simulink model "P702_NI_SoftECU"  (R2019a)
settings: Solver=ode1  StartTime=0.0  StopTime=Inf  FixedStep=0.001  RelTol=1e-3  EnableMultiTasking=on
PreLoadFcn:
  | run '.\VeriStand_BlockSet\NIVeriStandAddPaths.m'
undefined symbols (not defined in the file or in its folder): magnitude
libraries: simulink x83, simulink_extras x1
(part 69 of 76)

== system P702_NI_SoftECU/Output/Subsystem2/To_NI_HIL/Soft_SCCM/Steering_Data ==
  AccButtnGapDecPress : Constant  Value=0
  AccButtnGapIncPress : Constant  Value=0
  AhbStat_B_Dsply : Constant  Value=0
  AslButtnOnOffCnclPress : Constant  Value=0
  AslButtnOnOffPress : Constant  Value=0
  CcAslButtnCnclPress : Constant  Value=0
  CcAslButtnCnclResPress : Constant  Value=0
  CcAslButtnOnPress : Constant  Value=0
  CcAslButtnResDecPress : Constant  Value=0
  CcAslButtnResIncPress : Constant  Value=0
  CcAslButtnSetDecPress : Constant  Value=0
  CcAslButtnSetIncPress : Constant  Value=0
  CcAslButtnSetPress : Constant  Value=0
  CcAsllButtnResPress : Constant  Value=0
  CcButtnOffPress : Constant  Value=0
  CcButtnOnOffCnclPress : Constant  Value=0
  CcButtnOnOffPress : Constant  Value=0
  CcButtnOnPress : Constant  Value=0
  HeadLghtHiCtrl_D_RqAhb : Constant  Value=0
  HeadLghtHiOn_B_StatAhb : Constant  Value=0
  bus_creator : BusCreator  Inputs=20
  out_port : Outport
  wires:
  bus_creator/1 -> out_port/1  "Subsystem2"
  AhbStat_B_Dsply/1 -> bus_creator/1  "AhbStat_B_Dsply"
  HeadLghtHiCtrl_D_RqAhb/1 -> bus_creator/2  "HeadLghtHiCtrl_D_RqAhb"
  HeadLghtHiOn_B_StatAhb/1 -> bus_creator/3  "HeadLghtHiOn_B_StatAhb"
  CcButtnOnPress/1 -> bus_creator/4  "CcButtnOnPress"
  CcButtnOffPress/1 -> bus_creator/5  "CcButtnOffPress"
  CcAslButtnCnclPress/1 -> bus_creator/6  "CcAslButtnCnclPress"
  CcAsllButtnResPress/1 -> bus_creator/7  "CcAsllButtnResPress"
  CcAslButtnResIncPress/1 -> bus_creator/8  "CcAslButtnResIncPress"
  CcAslButtnSetIncPress/1 -> bus_creator/9  "CcAslButtnSetIncPress"
  CcAslButtnSetDecPress/1 -> bus_creator/10  "CcAslButtnSetDecPress"
  CcAslButtnSetPress/1 -> bus_creator/11  "CcAslButtnSetPress"
  AccButtnGapIncPress/1 -> bus_creator/12  "AccButtnGapIncPress"
  AccButtnGapDecPress/1 -> bus_creator/13  "AccButtnGapDecPress"
  AslButtnOnOffPress/1 -> bus_creator/14  "AslButtnOnOffPress"
  AslButtnOnOffCnclPress/1 -> bus_creator/15  "AslButtnOnOffCnclPress"
  CcButtnOnOffPress/1 -> bus_creator/16  "CcButtnOnOffPress"
  CcButtnOnOffCnclPress/1 -> bus_creator/17  "CcButtnOnOffCnclPress"
  CcAslButtnResDecPress/1 -> bus_creator/18  "CcAslButtnResDecPress"
  CcAslButtnOnPress/1 -> bus_creator/19  "CcAslButtnOnPress"
  CcAslButtnCnclResPress/1 -> bus_creator/20  "CcAslButtnCnclResPress"

== system P702_NI_SoftECU/Output/Subsystem2/To_NI_HIL/Soft_SCCM/Steering_Wheel_Data2 ==
  SteWhlSwtchBack_B_Stat : Constant  Value=0
  SteWhlSwtchDown_B_Stat : Constant  Value=0
  SteWhlSwtchLeft_B_Stat : Constant  Value=0
  SteWhlSwtchMenu_B_Stat : Constant  Value=0
  SteWhlSwtchOk_B_Stat : Constant  Value=0
  SteWhlSwtchRght_B_Stat : Constant  Value=0
  SteWhlSwtchUp_B_Stat : Constant  Value=0
  bus_creator : BusCreator  Inputs=7
  out_port : Outport
  wires:
  bus_creator/1 -> out_port/1  "Subsystem2"
  SteWhlSwtchOk_B_Stat/1 -> bus_creator/1  "SteWhlSwtchOk_B_Stat"
  SteWhlSwtchUp_B_Stat/1 -> bus_creator/2  "SteWhlSwtchUp_B_Stat"
  SteWhlSwtchDown_B_Stat/1 -> bus_creator/3  "SteWhlSwtchDown_B_Stat"
  SteWhlSwtchLeft_B_Stat/1 -> bus_creator/4  "SteWhlSwtchLeft_B_Stat"
  SteWhlSwtchRght_B_Stat/1 -> bus_creator/5  "SteWhlSwtchRght_B_Stat"
  SteWhlSwtchMenu_B_Stat/1 -> bus_creator/6  "SteWhlSwtchMenu_B_Stat"
  SteWhlSwtchBack_B_Stat/1 -> bus_creator/7  "SteWhlSwtchBack_B_Stat"

== system P702_NI_SoftECU/Output/Subsystem2/To_NI_HIL/Soft_TCM/TransGearData ==
  GearLvrPos_D_Actl : Constant  Value=0
  bus_creator : BusCreator  Inputs=1
  out_port : Outport
  wires:
  bus_creator/1 -> out_port/1  "Subsystem2"
  GearLvrPos_D_Actl/1 -> bus_creator/1  "GearLvrPos_D_Actl"

== system P702_NI_SoftECU/SoftECU/ABS/Logic/Wheel Direction/If Action Subsystem1 ==
  In1 : Inport
  Action Port : ActionPort  ActionPortLabel=if { }
  Out1 : Outport
  wires:
  In1/1 -> Out1/1

== system P702_NI_SoftECU/SoftECU/ABS/Logic/Wheel Direction/If Action Subsystem2 ==
  In1 : Inport
  Action Port : ActionPort  ActionPortLabel=elseif { }
  Out1 : Outport
  wires:
  In1/1 -> Out1/1

== system P702_NI_SoftECU/SoftECU/ABS/Logic/Wheel Direction/If Action Subsystem3 ==
  In1 : Inport
  Action Port : ActionPort  ActionPortLabel=elseif { }
  Out1 : Outport
  wires:
  In1/1 -> Out1/1

== system P702_NI_SoftECU/SoftECU/ABS/Logic/Wheel Direction/If Action Subsystem4 ==
  In1 : Inport
  Action Port : ActionPort  ActionPortLabel=if { }
  Out1 : Outport
  wires:
  In1/1 -> Out1/1

== system P702_NI_SoftECU/SoftECU/ABS/Logic/Wheel Direction/If Action Subsystem5 ==
  In1 : Inport
  Action Port : ActionPort  ActionPortLabel=elseif { }
  Out1 : Outport
  wires:
  In1/1 -> Out1/1

== system P702_NI_SoftECU/SoftECU/ABS/Logic/Wheel Direction/If Action Subsystem6 ==
  In1 : Inport
  Action Port : ActionPort  ActionPortLabel=elseif { }
  Out1 : Outport
  wires:
  In1/1 -> Out1/1

== system P702_NI_SoftECU/SoftECU/BCM/Logic/IgnitionState/If Action Subsystem1 ==
  In1 : Inport
  Action Port : ActionPort  ActionPortLabel=if { }
  Out1 : Outport
  wires:
  In1/1 -> Out1/1

== system P702_NI_SoftECU/SoftECU/BCM/Logic/IgnitionState/If Action Subsystem2 ==
  In1 : Inport
  Action Port : ActionPort  ActionPortLabel=elseif { }
  Out1 : Outport
  wires:
  In1/1 -> Out1/1

== system P702_NI_SoftECU/SoftECU/BCM/Logic/IgnitionState/If Action Subsystem3 ==
  In1 : Inport
  Action Port : ActionPort  ActionPortLabel=elseif { }
  Out1 : Outport
  wires:
  In1/1 -> Out1/1

== system P702_NI_SoftECU/SoftECU/BCM/Logic/IgnitionState/If Action Subsystem4 ==
  In1 : Inport
  Action Port : ActionPort  ActionPortLabel=elseif { }
  Out1 : Outport
  wires:
  In1/1 -> Out1/1

== system P702_NI_SoftECU/SoftECU/BCM/Logic/IgnitionState/If Action Subsystem5 ==
  In1 : Inport
  Action Port : ActionPort  ActionPortLabel=else { }
  Out1 : Outport
  wires:
  In1/1 -> Out1/1

== system P702_NI_SoftECU/SoftECU/BCM/Logic/OdometerValues/If Action Subsystem1 ==
  In1 : Inport
  Action Port : ActionPort  ActionPortLabel=if { }
  Out1 : Outport
  wires:
  In1/1 -> Out1/1

== system P702_NI_SoftECU/SoftECU/BCM/Logic/OdometerValues/If Action Subsystem4 ==
  In1 : Inport
  Action Port : ActionPort  ActionPortLabel=else { }
  Out1 : Outport
  wires:
  In1/1 -> Out1/1

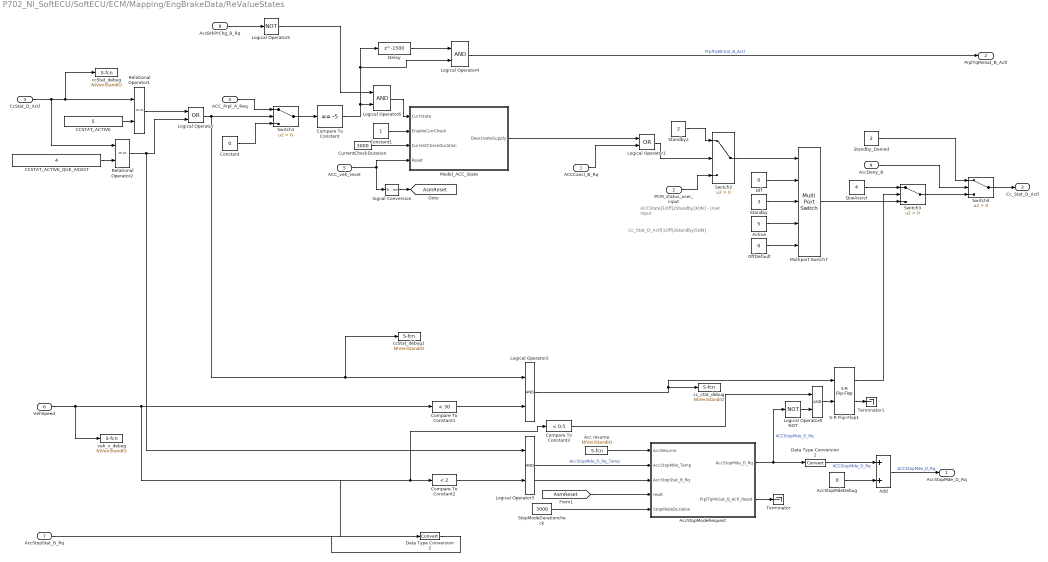
== system P702_NI_SoftECU/SoftECU/ECM/Mapping/EngBrakeData/ReValueStates ==
  note: ACCState[1Off|2Standby|3ON] -
      | User Input
  note: Cc_Stat_D_Actl[1Off|3Standby|5ON]
  ACCCancl_B_Rq : Inport
  PCM_status_user_input : Inport  Port=2
  CcStat_D_Actl : Inport  Port=3
  ACC_Prpl_A_Req : Inport  Port=4
  ACC_veh_reset : Inport  Port=5
  VehSpeed : Inport  Port=6
  AccStopStat_B_Rq : Inport  Port=7
  AccBrkPrChg_B_Rq : Inport  Port=8
  AccDeny_B : Inport  Port=9  OutDataTypeStr=boolean
  Acc resume : S-Function  Priority=1  FunctionName=NIVeriStandIO  Parameters=width dtype portnum stime stype btype  SFunctionDeploymentMode=off  EnableBusSupport=off  mask(NI VeriStand Inport){portnum=1, width=-1, stime=-1, dtype=auto, stype=auto, btype=1}
      mask prompts: portnum "Port number:"; width "Port dimensions (-1 for dynamically sized):"; stime "Sample time (-1 for inherited):"; dtype "Data type:"; stype "Signal type:"; btype "Block type:"
      mask help: Use this inport on any level of nested subsystems to allow NI VeriStand software to map signals to it.
      mask init:
      | NIVeriStandIO_init;
      settings: CopyFcn=NIVeriStand_MDL_functions('', 'IO_copy');  DeleteFcn=NIVeriStand_MDL_functions('', 'IO_delete');  MoveFcn=set_param(gcb, 'Mask', 'on');
      mask Callback portnum: NIVeriStand_MDL_functions('', 'IO_setportnum');
      mask TypeOptions dtype: auto | double | single | int8 | uint8 | int16 | uint16 | int32 | uint32 | boolean
      mask Callback dtype: NIVeriStand_MDL_functions('', 'IO_booleansignal');
      mask TypeOptions stype: auto | real | complex
      mask Display:
      | patch([-x x], [-y y], [.90980 .81960 .32156]);
      | plot([xrad -x x xrad], [yrad -y y yrad]);
      | fprintf('NI In%d', portnum);
  AccStopMdeDebug : Constant  Value=0
  AccStopModeRequest : Stateflow chart  TreatAsAtomicUnit=on
  Active : Constant  Value=5
  Add : Sum  OutDataTypeStr=double
  CCSTAT_ACTIVE : Constant  Description=_V1P2R1PX.CMM.000_81_  Value=5
  CCSTAT_ACTIVE_QUE_ASSIST : Constant  Description=_V1P2R1PX.CMM.000_82_  Value=4
  Compare To Constant : simulink/Logic and Bit Operations/Compare To Constant  relop===  const=-5  OutDataTypeStr=boolean
  Compare To Constant1 : simulink/Logic and Bit Operations/Compare To Constant  relop=<  const=30  OutDataTypeStr=boolean
  Compare To Constant2 : simulink/Logic and Bit Operations/Compare To Constant  relop=<  const=2  OutDataTypeStr=boolean
  Compare To Constant3 : simulink/Logic and Bit Operations/Compare To Constant  relop=<  const=0.5  OutDataTypeStr=boolean
  Constant : Constant  Value=0
  Constant1 : Constant
  CurrentCheckDuration : Constant  Value=3000  OutDataTypeStr=double
  Data Type Conversion1 : DataTypeConversion
  Data Type Conversion2 : DataTypeConversion
  Delay : Delay  DelayLength=1500
  Logical Operator : Logic  Description=_V1P2R1PX.CMM.000_84_  Operator=OR  AllPortsSameDT=off  OutDataTypeStr=boolean
  Logical Operator1 : Logic  Operator=OR  AllPortsSameDT=off  OutDataTypeStr=boolean
  Logical Operator2 : Logic  IconShape=distinctive  AllPortsSameDT=off  OutDataTypeStr=boolean
  Logical Operator3 : Logic  IconShape=distinctive  AllPortsSameDT=off  OutDataTypeStr=boolean
  Logical Operator4 : Logic  AllPortsSameDT=off  OutDataTypeStr=boolean
  Logical Operator5 : Logic  Operator=NOT  AllPortsSameDT=off  OutDataTypeStr=boolean
  Logical Operator6 : Logic  AllPortsSameDT=off  OutDataTypeStr=boolean
  Logical Operator8 : Logic  IconShape=distinctive  AllPortsSameDT=off  OutDataTypeStr=boolean
  Model_ACC_State : Stateflow chart  TreatAsAtomicUnit=on
  Multiport Switch7 : MultiPortSwitch  DataPortForDefault=Additional data port  SaturateOnIntegerOverflow=on
  NOT : Logic  Operator=NOT  IconShape=distinctive  AllPortsSameDT=off  OutDataTypeStr=boolean
  Off : Constant  Value=0
  OffDefault : Constant  Value=0
  QueAssist : Constant  Value=4
  Relational Operator1 : RelationalOperator  Description=_V1P2R1PX.CMM.000_85_  Operator===  OutDataTypeStr=boolean  RndMeth=Nearest
  Relational Operator2 : RelationalOperator  Description=_V1P2R1PX.CMM.000_86_  Operator===  OutDataTypeStr=boolean  RndMeth=Nearest
  S-R Flip-Flop1 : simulink_extras/Flip Flops/S-R Flip-Flop  initial_condition=0
  Signal Conversion : SignalConversion  OverrideOpt=off
  Standby : Constant  Value=3
  Standby2 : Constant  Value=2
  "Standby_Denied " : Constant  Value=2
  StopModeDurationcheck : Constant  Value=3000  OutDataTypeStr=uint16
  Switch{1..4} (4 alike) : Switch  Criteria=u2 > Threshold
  Terminator : Terminator
  Terminator1 : Terminator
  ccStat_debug : S-Function  Priority=3  FunctionName=NIVeriStandIO  Parameters=width dtype portnum stime stype btype  SFunctionDeploymentMode=off  EnableBusSupport=off  mask(NI VeriStand Outport){portnum=3, width=-1, stime=-1, dtype=auto, stype=auto, btype=0}
      mask prompts: portnum "Port number:"; width "Port dimensions (-1 for dynamically sized):"; stime "Sample time (-1 for inherited):"; dtype "Data type:"; stype "Signal type:"; btype "Block type:"
      mask help: Use this outport on any level of nested subsystems to allow NI VeriStand software to map signals to it.
      mask init:
      | NIVeriStandIO_init;
      settings: CopyFcn=NIVeriStand_MDL_functions('', 'IO_copy');  DeleteFcn=NIVeriStand_MDL_functions('', 'IO_delete');  MoveFcn=set_param(gcb, 'Mask', 'on');
      mask Callback portnum: NIVeriStand_MDL_functions('', 'IO_setportnum');
      mask TypeOptions dtype: auto | double | single | int8 | uint8 | int16 | uint16 | int32 | uint32 | boolean
      mask Callback dtype: NIVeriStand_MDL_functions('', 'IO_booleansignal');
      mask TypeOptions stype: auto | real | complex
      mask Display:
      | patch([-x x], [-y y], [.90980 .81960 .32156]);
      | plot([xrad -x x xrad], [yrad -y y yrad]);
      | fprintf('NI Out%d', portnum);
  ccStat_debug1 : S-Function  Priority=4  FunctionName=NIVeriStandIO  Parameters=width dtype portnum stime stype btype  SFunctionDeploymentMode=off  EnableBusSupport=off  mask(NI VeriStand Outport){portnum=4, width=-1, stime=-1, dtype=auto, stype=auto, btype=0}
      mask prompts: portnum "Port number:"; width "Port dimensions (-1 for dynamically sized):"; stime "Sample time (-1 for inherited):"; dtype "Data type:"; stype "Signal type:"; btype "Block type:"
      mask help: Use this outport on any level of nested subsystems to allow NI VeriStand software to map signals to it.
      mask init:
      | NIVeriStandIO_init;
      settings: CopyFcn=NIVeriStand_MDL_functions('', 'IO_copy');  DeleteFcn=NIVeriStand_MDL_functions('', 'IO_delete');  MoveFcn=set_param(gcb, 'Mask', 'on');
      mask Callback portnum: NIVeriStand_MDL_functions('', 'IO_setportnum');
      mask TypeOptions dtype: auto | double | single | int8 | uint8 | int16 | uint16 | int32 | uint32 | boolean
      mask Callback dtype: NIVeriStand_MDL_functions('', 'IO_booleansignal');
      mask TypeOptions stype: auto | real | complex
      mask Display:
      | patch([-x x], [-y y], [.90980 .81960 .32156]);
      | plot([xrad -x x xrad], [yrad -y y yrad]);
      | fprintf('NI Out%d', portnum);
  cc_stat_debug : S-Function  Priority=1  FunctionName=NIVeriStandIO  Parameters=width dtype portnum stime stype btype  SFunctionDeploymentMode=off  EnableBusSupport=off  mask(NI VeriStand Outport){portnum=1, width=-1, stime=-1, dtype=auto, stype=auto, btype=0}
      mask prompts: portnum "Port number:"; width "Port dimensions (-1 for dynamically sized):"; stime "Sample time (-1 for inherited):"; dtype "Data type:"; stype "Signal type:"; btype "Block type:"
      mask help: Use this outport on any level of nested subsystems to allow NI VeriStand software to map signals to it.
      mask init:
      | NIVeriStandIO_init;
      settings: CopyFcn=NIVeriStand_MDL_functions('', 'IO_copy');  DeleteFcn=NIVeriStand_MDL_functions('', 'IO_delete');  MoveFcn=set_param(gcb, 'Mask', 'on');
      mask Callback portnum: NIVeriStand_MDL_functions('', 'IO_setportnum');
      mask TypeOptions dtype: auto | double | single | int8 | uint8 | int16 | uint16 | int32 | uint32 | boolean
      mask Callback dtype: NIVeriStand_MDL_functions('', 'IO_booleansignal');
      mask TypeOptions stype: auto | real | complex
      mask Display:
      | patch([-x x], [-y y], [.90980 .81960 .32156]);
      | plot([xrad -x x xrad], [yrad -y y yrad]);
      | fprintf('NI Out%d', portnum);
  veh_v_debug : S-Function  Priority=2  FunctionName=NIVeriStandIO  Parameters=width dtype portnum stime stype btype  SFunctionDeploymentMode=off  EnableBusSupport=off  mask(NI VeriStand Outport){portnum=2, width=-1, stime=-1, dtype=auto, stype=auto, btype=0}
      mask prompts: portnum "Port number:"; width "Port dimensions (-1 for dynamically sized):"; stime "Sample time (-1 for inherited):"; dtype "Data type:"; stype "Signal type:"; btype "Block type:"
      mask help: Use this outport on any level of nested subsystems to allow NI VeriStand software to map signals to it.
      mask init:
      | NIVeriStandIO_init;
      settings: CopyFcn=NIVeriStand_MDL_functions('', 'IO_copy');  DeleteFcn=NIVeriStand_MDL_functions('', 'IO_delete');  MoveFcn=set_param(gcb, 'Mask', 'on');
      mask Callback portnum: NIVeriStand_MDL_functions('', 'IO_setportnum');
      mask TypeOptions dtype: auto | double | single | int8 | uint8 | int16 | uint16 | int32 | uint32 | boolean
      mask Callback dtype: NIVeriStand_MDL_functions('', 'IO_booleansignal');
      mask TypeOptions stype: auto | real | complex
      mask Display:
      | patch([-x x], [-y y], [.90980 .81960 .32156]);
      | plot([xrad -x x xrad], [yrad -y y yrad]);
      | fprintf('NI Out%d', portnum);
  AccStopMde_D_Rq : Outport
  PrplTqMnSat_B_Actl : Outport  Port=2
  Cc_Stat_D_Actl : Outport  Port=3
  tag scope: AsmReset=global
  wires:
  PCM_status_user_input/1 -> Switch2/3
  ACCCancl_B_Rq/1 -> Logical Operator1/2
  Relational Operator1/1 -> Logical Operator/1
  CCSTAT_ACTIVE_QUE_ASSIST/1 -> Relational Operator2/2
  CCSTAT_ACTIVE/1 -> Relational Operator1/2
  CcStat_D_Actl/1 -> Relational Operator2/1, ccStat_debug/1, Relational Operator1/1
  ACC_Prpl_A_Req/1 -> Switch1/1
  Constant/1 -> Switch1/3
  Constant1/1 -> Model_ACC_State/2(EnableCurrCheck)
  CurrentCheckDuration/1 -> Model_ACC_State/3(CurrentCheckDuration)
  Model_ACC_State/1(DeactivateSupply) -> Logical Operator1/1
  Standby2/1 -> Switch2/1
  Logical Operator1/1 -> Switch2/2
  StopModeDurationcheck/1 -> AccStopModeRequest/5(StopModeDuration)
  Logical Operator/1 -> ccStat_debug1/1, Logical Operator2/1, Switch1/2
  Compare To Constant1/1 -> Logical Operator2/2
  Relational Operator2/1 -> Logical Operator3/1, Logical Operator/2
  [AsmReset] -> AccStopModeRequest/4(reset)
  Compare To Constant2/1 -> Logical Operator3/2
  AccStopStat_B_Rq/1 -> Data Type Conversion2/1
  Logical Operator3/1 -> AccStopModeRequest/2(AccStopMde_Temp)  "AccStopMde_D_Rq_Temp"
  Signal Conversion/1 -> [AsmReset]
  ACC_veh_reset/1 -> Signal Conversion/1, Model_ACC_State/4(Reset)
  AccBrkPrChg_B_Rq/1 -> Logical Operator5/1
  Delay/1 -> Logical Operator4/1
  Compare To Constant/1 -> Delay/1, Logical Operator4/2, Logical Operator6/2
  Logical Operator6/1 -> Model_ACC_State/1(CurrState)
  Logical Operator5/1 -> Logical Operator6/1
  AccStopModeRequest/1(AccStopMde_D_Rq) -> Data Type Conversion1/1, NOT/1  "ACCStopMde_D_Rq"
  Add/1 -> AccStopMde_D_Rq/1  "ACCStopMde_D_Rq"
  Data Type Conversion2/1 -> AccStopModeRequest/3(AccStopStat_B_Rq)
  Data Type Conversion1/1 -> Add/1  "ACCStopMde_D_Rq"
  AccStopMdeDebug/1 -> Add/2
  Logical Operator4/1 -> PrplTqMnSat_B_Actl/1  "PrplTqMnSat_B_Actl"
  AccStopModeRequest/2(PrplTqMnSat_B_Actl_Reset) -> Terminator/1
  Logical Operator2/1 -> S-R Flip-Flop1/1, cc_stat_debug/1
  S-R Flip-Flop1/2 -> Terminator1/1
  Logical Operator8/1 -> S-R Flip-Flop1/2
  NOT/1 -> Logical Operator8/2
  Compare To Constant3/1 -> Logical Operator8/1
  Acc resume/1 -> AccStopModeRequest/1(AccResume)
  VehSpeed/1 -> veh_v_debug/1, Compare To Constant3/1, Compare To Constant2/1, Compare To Constant1/1
  Switch1/1 -> Compare To Constant/1
  Active/1 -> Multiport Switch7/4
  Standby/1 -> Multiport Switch7/3
  Off/1 -> Multiport Switch7/2
  Switch2/1 -> Multiport Switch7/1
  S-R Flip-Flop1/1 -> Switch3/2
  QueAssist/1 -> Switch3/1
  Multiport Switch7/1 -> Switch3/3
  Switch3/1 -> Switch4/3
  AccDeny_B/1 -> Switch4/2
  Switch4/1 -> Cc_Stat_D_Actl/1
  "Standby_Denied "/1 -> Switch4/1
  OffDefault/1 -> Multiport Switch7/5

== system P702_NI_SoftECU/SoftECU/MRR/Logic/Bus2Array/Azimuth ==
  In1 : Inport
  Bus Selector2 : BusSelector  OutputSignals=CAN_DET_AZIMUTH_01[rad],CAN_DET_AZIMUTH_02[rad],CAN_DET_AZIMUTH_03[rad]
  Mux2 : Mux  Inputs=3
  Out1 : Outport
  wires:
  In1/1 -> Bus Selector2/1
  Bus Selector2/2 -> Mux2/2  "<CAN_DET_AZIMUTH_02[rad]>"
  Bus Selector2/3 -> Mux2/3  "<CAN_DET_AZIMUTH_03[rad]>"
  Bus Selector2/1 -> Mux2/1  "<CAN_DET_AZIMUTH_01[rad]>"
  Mux2/1 -> Out1/1

== system P702_NI_SoftECU/SoftECU/MRR/Logic/Bus2Array/Range ==
  In1 : Inport
  Bus Selector2 : BusSelector  OutputSignals=CAN_DET_RANGE_01[m],CAN_DET_RANGE_02[m],CAN_DET_RANGE_03[m]
  Mux2 : Mux  Inputs=3
  Out1 : Outport
  wires:
  In1/1 -> Bus Selector2/1
  Bus Selector2/2 -> Mux2/2  "<CAN_DET_RANGE_02[m]>"
  Bus Selector2/3 -> Mux2/3  "<CAN_DET_RANGE_03[m]>"
  Bus Selector2/1 -> Mux2/1  "<CAN_DET_RANGE_01[m]>"
  Mux2/1 -> Out1/1

== system P702_NI_SoftECU/SoftECU/MRR/Logic/Bus2Array/Range_Rate ==
  In1 : Inport
  Bus Selector2 : BusSelector  OutputSignals=CAN_DET_RANGE_RATE_01[m/s],CAN_DET_RANGE_RATE_02[m/s],CAN_DET_RANGE_RATE_03[m/s]
  Mux2 : Mux  Inputs=3
  Out1 : Outport
  wires:
  In1/1 -> Bus Selector2/1
  Bus Selector2/2 -> Mux2/2  "<CAN_DET_RANGE_RATE_02[m/s]>"
  Bus Selector2/3 -> Mux2/3  "<CAN_DET_RANGE_RATE_03[m/s]>"
  Bus Selector2/1 -> Mux2/1  "<CAN_DET_RANGE_RATE_01[m/s]>"
  Mux2/1 -> Out1/1

== system P702_NI_SoftECU/SoftECU/PCM/Logic1/EngVehSpeed/CalcGearRvrseActv ==
  note: default is not Confirmed
  In1 : Inport
  ActiveConfirmed : Constant  Value=3
  ActiveNotConfirmed : Constant  Value=2
  Add : Sum
  Constant : Constant  Value=2
  Constant1 : Constant  Value=0
  Constant2 : Constant
  Fault : Constant  Value=7
  Fault1 : Constant  Value=7
  InactiveConfirmed : Constant
  InactiveNotConfirmed1 : Constant  Value=0
  Multiport Switch : MultiPortSwitch  Inputs=7
  Multiport Switch1 : MultiPortSwitch  Inputs=7
  Multiport Switch2 : MultiPortSwitch  DataPortOrder=Zero-based contiguous  Inputs=2  zeroidx=on
  Terminator : Terminator
  Out1 : Outport
  wires:
  In1/1 -> Add/1  "ManGearAsm"
  Constant/1 -> Add/2
  ActiveConfirmed/1 -> Multiport Switch/2
  InactiveConfirmed/1 -> Multiport Switch/3, Multiport Switch/4, Multiport Switch/5, Multiport Switch/6, Multiport Switch/7
  Fault/1 -> Multiport Switch/8
  ActiveNotConfirmed/1 -> Multiport Switch1/2
  InactiveNotConfirmed1/1 -> Multiport Switch1/7, Multiport Switch1/6, Multiport Switch1/5, Multiport Switch1/4, Multiport Switch1/3
  Fault1/1 -> Multiport Switch1/8
  Constant1/1 -> Multiport Switch2/1
  Multiport Switch2/1 -> Terminator/1  "GearRvrseActv_B_Actl"
  Add/1 -> Multiport Switch1/1, Multiport Switch/1
  Multiport Switch1/1 -> Multiport Switch2/2
  Multiport Switch/1 -> Multiport Switch2/3
  Constant2/1 -> Out1/1

== system P702_NI_SoftECU/SoftECU/PCM/Logic1/Key/PowerStates ==
  In1 : Inport
  In2 : Inport  Port=2
  In3 : Inport  Port=3
  AndRunstartWithBatterySw : Logic  AllPortsSameDT=off  OutDataTypeStr=boolean
  BatterySwitch_B : Constant
  Bus Creator4 : BusCreator  Inputs=5
  Gain{,1..3} (4 alike) : Gain
  RunStartRlyExt_B : Constant
  SelectKV : Switch  Criteria=u2 > Threshold
  SelectKV1 : Switch  Criteria=u2 > Threshold
  Subsystem1 : Subsystem
  Out1 : Outport
  wires:
  In1/1 -> Subsystem1/1(No_KeyPostn)
  Gain3/1 -> Bus Creator4/4  "IgnSwtchKeyIn_B"
  Gain2/1 -> Bus Creator4/3  "VehTe75_B"
  Gain1/1 -> SelectKV1/3  "VehTe15_B"
  Gain/1 -> SelectKV/3  "VehTe50Rly_B"
  Bus Creator4/1 -> Out1/1
  Subsystem1/4(KeyIn_B) -> Gain3/1  "IgnSwtchKeyIn_B"
  Subsystem1/3(Te75_B) -> Gain2/1  "DrvTe75_B"
  Subsystem1/2(Te15_B) -> Gain1/1  "DrvTe15_B"
  Subsystem1/1(Te50_B) -> Gain/1  "DrvTe50_B"
  In3/1 -> SelectKV/2, Bus Creator4/5, SelectKV1/2  "KvActive"
  SelectKV/1 -> Bus Creator4/1  "VehTe50Rly_B"
  In2/1 -> SelectKV/1  "VehTe50Rly_B"
  AndRunstartWithBatterySw/1 -> SelectKV1/1  "VehTe15_B"
  BatterySwitch_B/1 -> AndRunstartWithBatterySw/1, Subsystem1/2(BatterySwitch_B)  "<BatterySwitch_B>"
  RunStartRlyExt_B/1 -> AndRunstartWithBatterySw/2  "<RunStartRlyExt_B>"
  SelectKV1/1 -> Bus Creator4/2  "VehTe15_B"

== system P702_NI_SoftECU/SoftECU/PCM/Logic1/Key/Start//Stop_Pulsing ==
  In1 : Inport
  Compare To Constant1 : simulink/Logic and Bit Operations/Compare To Constant  relop===  const=3  OutDataTypeStr=uint8
  Compare To Constant2 : simulink/Logic and Bit Operations/Compare To Constant  relop===  const=2  OutDataTypeStr=uint8
  Compare To Constant3 : simulink/Logic and Bit Operations/Compare To Constant  relop===  const=1  OutDataTypeStr=uint8
  Data Type Conversion2 : DataTypeConversion
  Data Type Conversion3 : DataTypeConversion
  Logical Operator1 : Logic  Operator=OR  Inputs=3  AllPortsSameDT=off  OutDataTypeStr=boolean
  Out1 : Outport
  wires:
  Data Type Conversion3/1 -> Logical Operator1/2
  Data Type Conversion2/1 -> Logical Operator1/1
  Compare To Constant2/1 -> Data Type Conversion2/1
  Compare To Constant3/1 -> Data Type Conversion3/1
  Logical Operator1/1 -> Out1/1
  In1/1 -> Compare To Constant2/1, Compare To Constant3/1, Compare To Constant1/1
  Compare To Constant1/1 -> Logical Operator1/3

== system P702_NI_SoftECU/SoftECU/PCM/Logic1/PrplWhlTot2Calc/GetTransmissionRatio ==
  Gear[-] : Inport
  Act_Gear_ratio : MultiPortSwitch  Inputs=8
  Act_Trans_ratio : MultiPortSwitch  Inputs=8
  AddOffset_for_R-N_gears : Sum
  Gear-ratio_mult_Trans-ratio : Product  RndMeth=Zero
  Offset_for_R-N_gears : Constant  Value=2
  gear_1 : Constant  Value=3.583
  gear_1-4_Trans : Constant  Value=4.067
  gear_2 : Constant  Value=1.952
  gear_3 : Constant  Value=1.194
  gear_4 : Constant  Value=0.842
  gear_5 : Constant  Value=0.943
  gear_5-6_Trans : Constant  Value=2.905
  gear_6 : Constant  Value=0.789
  gear_N : Constant  Value=0
  gear_N_Trans : Constant  Value=0
  gear_R : Constant  Value=2.167
  gear_R_Trans : Constant  Value=2.905
  Transmission_Ratio[-] : Outport
  wires:
  Gear[-]/1 -> AddOffset_for_R-N_gears/1
  gear_N/1 -> Act_Gear_ratio/3
  gear_1/1 -> Act_Gear_ratio/4
  gear_2/1 -> Act_Gear_ratio/5
  gear_3/1 -> Act_Gear_ratio/6
  gear_4/1 -> Act_Gear_ratio/7
  gear_5/1 -> Act_Gear_ratio/8
  gear_6/1 -> Act_Gear_ratio/9
  gear_5-6_Trans/1 -> Act_Trans_ratio/8, Act_Trans_ratio/9
  gear_1-4_Trans/1 -> Act_Trans_ratio/4, Act_Trans_ratio/5, Act_Trans_ratio/6, Act_Trans_ratio/7
  gear_N_Trans/1 -> Act_Trans_ratio/3
  gear_R/1 -> Act_Gear_ratio/2
  gear_R_Trans/1 -> Act_Trans_ratio/2
  Offset_for_R-N_gears/1 -> AddOffset_for_R-N_gears/2
  AddOffset_for_R-N_gears/1 -> Act_Gear_ratio/1, Act_Trans_ratio/1
  Act_Gear_ratio/1 -> Gear-ratio_mult_Trans-ratio/2
  Gear-ratio_mult_Trans-ratio/1 -> Transmission_Ratio[-]/1
  Act_Trans_ratio/1 -> Gear-ratio_mult_Trans-ratio/1

== system P702_NI_SoftECU/SoftECU/PCM/Logic1/Speed_Accel_Controller/ACC_Accel_Controller ==
  Vehicle_Ax : Inport
  Desried_accel : Inport  Port=2
  Abs : Abs
  Add : Sum  Inputs=-+
  Gain : Gain  Gain=1.5
  Gain1 : Gain  Gain=0.5
  Gain2 : Gain  Gain=0
  Saturation : Saturate  UpperLimit=20  LowerLimit=0
  Saturation1 : Saturate  UpperLimit=0  LowerLimit=-10
  Throttle_Pos : Outport
  Brake_MS_Pressure : Outport  Port=2
  wires:
  Abs/1 -> Gain1/1
  Gain1/1 -> Brake_MS_Pressure/1
  Gain/1 -> Saturation/1
  Saturation1/1 -> Abs/1
  Saturation/1 -> Throttle_Pos/1
  Vehicle_Ax/1 -> Gain2/1
  Gain2/1 -> Add/1
  Desried_accel/1 -> Add/2
  Add/1 -> Saturation1/1, Gain/1

== system P702_NI_SoftECU/SoftECU/PCM/Logic1/Speed_Accel_Controller/Speed_Controller ==
  Veh_Spd : Inport
  Desried_Spd : Inport  Port=2
  Abs : Abs
  Abs1 : Abs
  Add : Sum  Inputs=+-
  Add1 : Sum  Inputs=+++
  Constant : Constant  Value=5
  Divide : Product  Inputs=**
  Divide1 : Product  Inputs=**
  Divide2 : Product  Inputs=**
  Divide3 : Product  Inputs=***
  Gain : Gain
  Gain1 : Gain  Gain=2
  Integrator : Integrator  ExternalReset=level
  KI : Constant  Value=0.5
  KP : Constant  Value=0.1
  KP3 : Constant  Value=0.1
  Relational Operator : RelationalOperator  Operator=>  OutDataTypeStr=boolean  RndMeth=Simplest
  Saturation : Saturate  UpperLimit=20  LowerLimit=0
  Saturation1 : Saturate  UpperLimit=0  LowerLimit=-5
  Throttle_Pos : Outport
  Brake_MS_Pressure : Outport  Port=2
  wires:
  Veh_Spd/1 -> [Vx]
  Desried_Spd/1 -> [Vtarget]
  [Vtarget] -> Add/1
  [Vx] -> Add/2
  Add/1 -> [Verr]
  KP/1 -> [KP]
  KI/1 -> [KI]
  KP3/1 -> [KP3]
  Divide/1 -> Add1/1
  Divide1/1 -> Add1/2
  Divide2/1 -> Add1/3
  [KP] -> Divide/2
  [KI] -> Divide1/2
  [KP3] -> Divide2/2
  [Verr] -> Divide3/1, Divide3/2, Divide3/3, Divide/1
  [Ierr] -> Divide1/1
  Divide3/1 -> Divide2/1
  Add1/1 -> Saturation1/1, Gain/1
  Gain/1 -> Saturation/1
  Saturation/1 -> Throttle_Pos/1
  Saturation1/1 -> Abs/1
  Gain1/1 -> Brake_MS_Pressure/1
  Abs/1 -> Gain1/1
  Integrator/1 -> [Ierr]
  [Verr] -> Integrator/1
  [Verr] -> Abs1/1
  Abs1/1 -> Relational Operator/1
  Constant/1 -> Relational Operator/2
  Relational Operator/1 -> Integrator/2

== system P702_NI_SoftECU/SoftECU/PCM/Logic1/States/Subsystem1 ==
  In1 : Inport
  Out1 : Outport
  wires:
  In1/1 -> Out1/1

== system P702_NI_SoftECU/SoftECU/PCM/Logic1/States/Subsystem2 ==
  In1 : Inport
  Out1 : Outport
  wires:
  In1/1 -> Out1/1

== system P702_NI_SoftECU/SoftECU/PCM/Logic1/States/Subsystem3 ==
  In1 : Inport
  Out1 : Outport
  wires:
  In1/1 -> Out1/1

== system P702_NI_SoftECU/SoftECU/PCM/Logic1/States/Subsystem4 ==
  In1 : Inport
  Out1 : Outport
  wires:
  In1/1 -> Out1/1

== system P702_NI_SoftECU/SoftECU/PCM/Logic1/States/Subsystem5 ==
  In1 : Inport
  Out1 : Outport
  wires:
  In1/1 -> Out1/1

== system P702_NI_SoftECU/SoftECU/PCM/Logic1/States/Subsystem6 ==
  In1 : Inport
  Out1 : Outport
  wires:
  In1/1 -> Out1/1

== system P702_NI_SoftECU/SoftECU/PCM/Logic1/States/Subsystem7 ==
  In1 : Inport
  Out1 : Outport
  wires:
  In1/1 -> Out1/1

== system P702_NI_SoftECU/SoftECU/PCM/Logic1/States/Test_PCM_Input ==
  In1 : Inport
  In2 : Inport  Port=2
  In3 : Inport  Port=3
  In4 : Inport  Port=4
  In5 : Inport  Port=5
  In6 : Inport  Port=6
  Test_ClutchSW : S-Function  Priority=5  FunctionName=NIVeriStandIO  Parameters=width dtype portnum stime stype btype  SFunctionDeploymentMode=off  EnableBusSupport=off  mask(NI VeriStand Outport){portnum=5, width=-1, stime=-1, dtype=auto, stype=auto, btype=0}
      mask prompts: portnum "Port number:"; width "Port dimensions (-1 for dynamically sized):"; stime "Sample time (-1 for inherited):"; dtype "Data type:"; stype "Signal type:"; btype "Block type:"
      mask help: Use this outport on any level of nested subsystems to allow NI VeriStand software to map signals to it.
      mask init:
      | NIVeriStandIO_init;
      settings: CopyFcn=NIVeriStand_MDL_functions('', 'IO_copy');  DeleteFcn=NIVeriStand_MDL_functions('', 'IO_delete');  MoveFcn=set_param(gcb, 'Mask', 'on');
      mask Callback portnum: NIVeriStand_MDL_functions('', 'IO_setportnum');
      mask TypeOptions dtype: auto | double | single | int8 | uint8 | int16 | uint16 | int32 | uint32 | boolean
      mask Callback dtype: NIVeriStand_MDL_functions('', 'IO_booleansignal');
      mask TypeOptions stype: auto | real | complex
      mask Display:
      | patch([-x x], [-y y], [.90980 .81960 .32156]);
      | plot([xrad -x x xrad], [yrad -y y yrad]);
      | fprintf('NI Out%d', portnum);
  Test_KVactive : S-Function  Priority=4  FunctionName=NIVeriStandIO  Parameters=width dtype portnum stime stype btype  SFunctionDeploymentMode=off  EnableBusSupport=off  mask(NI VeriStand Outport){portnum=4, width=-1, stime=-1, dtype=auto, stype=auto, btype=0}
      mask prompts: portnum "Port number:"; width "Port dimensions (-1 for dynamically sized):"; stime "Sample time (-1 for inherited):"; dtype "Data type:"; stype "Signal type:"; btype "Block type:"
      mask help: Use this outport on any level of nested subsystems to allow NI VeriStand software to map signals to it.
      mask init:
      | NIVeriStandIO_init;
      settings: CopyFcn=NIVeriStand_MDL_functions('', 'IO_copy');  DeleteFcn=NIVeriStand_MDL_functions('', 'IO_delete');  MoveFcn=set_param(gcb, 'Mask', 'on');
      mask Callback portnum: NIVeriStand_MDL_functions('', 'IO_setportnum');
      mask TypeOptions dtype: auto | double | single | int8 | uint8 | int16 | uint16 | int32 | uint32 | boolean
      mask Callback dtype: NIVeriStand_MDL_functions('', 'IO_booleansignal');
      mask TypeOptions stype: auto | real | complex
      mask Display:
      | patch([-x x], [-y y], [.90980 .81960 .32156]);
      | plot([xrad -x x xrad], [yrad -y y yrad]);
      | fprintf('NI Out%d', portnum);
  Test_KeyPostn_No : S-Function  Priority=1  FunctionName=NIVeriStandIO  Parameters=width dtype portnum stime stype btype  SFunctionDeploymentMode=off  EnableBusSupport=off  mask(NI VeriStand Outport){portnum=1, width=-1, stime=-1, dtype=auto, stype=auto, btype=0}
      mask prompts: portnum "Port number:"; width "Port dimensions (-1 for dynamically sized):"; stime "Sample time (-1 for inherited):"; dtype "Data type:"; stype "Signal type:"; btype "Block type:"
      mask help: Use this outport on any level of nested subsystems to allow NI VeriStand software to map signals to it.
      mask init:
      | NIVeriStandIO_init;
      settings: CopyFcn=NIVeriStand_MDL_functions('', 'IO_copy');  DeleteFcn=NIVeriStand_MDL_functions('', 'IO_delete');  MoveFcn=set_param(gcb, 'Mask', 'on');
      mask Callback portnum: NIVeriStand_MDL_functions('', 'IO_setportnum');
      mask TypeOptions dtype: auto | double | single | int8 | uint8 | int16 | uint16 | int32 | uint32 | boolean
      mask Callback dtype: NIVeriStand_MDL_functions('', 'IO_booleansignal');
      mask TypeOptions stype: auto | real | complex
      mask Display:
      | patch([-x x], [-y y], [.90980 .81960 .32156]);
      | plot([xrad -x x xrad], [yrad -y y yrad]);
      | fprintf('NI Out%d', portnum);
  Test_PCMWakeup : S-Function  Priority=6  FunctionName=NIVeriStandIO  Parameters=width dtype portnum stime stype btype  SFunctionDeploymentMode=off  EnableBusSupport=off  mask(NI VeriStand Outport){portnum=6, width=-1, stime=-1, dtype=auto, stype=auto, btype=0}
      mask prompts: portnum "Port number:"; width "Port dimensions (-1 for dynamically sized):"; stime "Sample time (-1 for inherited):"; dtype "Data type:"; stype "Signal type:"; btype "Block type:"
      mask help: Use this outport on any level of nested subsystems to allow NI VeriStand software to map signals to it.
      mask init:
      | NIVeriStandIO_init;
      settings: CopyFcn=NIVeriStand_MDL_functions('', 'IO_copy');  DeleteFcn=NIVeriStand_MDL_functions('', 'IO_delete');  MoveFcn=set_param(gcb, 'Mask', 'on');
      mask Callback portnum: NIVeriStand_MDL_functions('', 'IO_setportnum');
      mask TypeOptions dtype: auto | double | single | int8 | uint8 | int16 | uint16 | int32 | uint32 | boolean
      mask Callback dtype: NIVeriStand_MDL_functions('', 'IO_booleansignal');
      mask TypeOptions stype: auto | real | complex
      mask Display:
      | patch([-x x], [-y y], [.90980 .81960 .32156]);
      | plot([xrad -x x xrad], [yrad -y y yrad]);
      | fprintf('NI Out%d', portnum);
  Test_Te15 : S-Function  Priority=3  FunctionName=NIVeriStandIO  Parameters=width dtype portnum stime stype btype  SFunctionDeploymentMode=off  EnableBusSupport=off  mask(NI VeriStand Outport){portnum=3, width=-1, stime=-1, dtype=auto, stype=auto, btype=0}
      mask prompts: portnum "Port number:"; width "Port dimensions (-1 for dynamically sized):"; stime "Sample time (-1 for inherited):"; dtype "Data type:"; stype "Signal type:"; btype "Block type:"
      mask help: Use this outport on any level of nested subsystems to allow NI VeriStand software to map signals to it.
      mask init:
      | NIVeriStandIO_init;
      settings: CopyFcn=NIVeriStand_MDL_functions('', 'IO_copy');  DeleteFcn=NIVeriStand_MDL_functions('', 'IO_delete');  MoveFcn=set_param(gcb, 'Mask', 'on');
      mask Callback portnum: NIVeriStand_MDL_functions('', 'IO_setportnum');
      mask TypeOptions dtype: auto | double | single | int8 | uint8 | int16 | uint16 | int32 | uint32 | boolean
      mask Callback dtype: NIVeriStand_MDL_functions('', 'IO_booleansignal');
      mask TypeOptions stype: auto | real | complex
      mask Display:
      | patch([-x x], [-y y], [.90980 .81960 .32156]);
      | plot([xrad -x x xrad], [yrad -y y yrad]);
      | fprintf('NI Out%d', portnum);
  Test_Te50 : S-Function  Priority=2  FunctionName=NIVeriStandIO  Parameters=width dtype portnum stime stype btype  SFunctionDeploymentMode=off  EnableBusSupport=off  mask(NI VeriStand Outport){portnum=2, width=-1, stime=-1, dtype=auto, stype=auto, btype=0}
      mask prompts: portnum "Port number:"; width "Port dimensions (-1 for dynamically sized):"; stime "Sample time (-1 for inherited):"; dtype "Data type:"; stype "Signal type:"; btype "Block type:"
      mask help: Use this outport on any level of nested subsystems to allow NI VeriStand software to map signals to it.
      mask init:
      | NIVeriStandIO_init;
      settings: CopyFcn=NIVeriStand_MDL_functions('', 'IO_copy');  DeleteFcn=NIVeriStand_MDL_functions('', 'IO_delete');  MoveFcn=set_param(gcb, 'Mask', 'on');
      mask Callback portnum: NIVeriStand_MDL_functions('', 'IO_setportnum');
      mask TypeOptions dtype: auto | double | single | int8 | uint8 | int16 | uint16 | int32 | uint32 | boolean
      mask Callback dtype: NIVeriStand_MDL_functions('', 'IO_booleansignal');
      mask TypeOptions stype: auto | real | complex
      mask Display:
      | patch([-x x], [-y y], [.90980 .81960 .32156]);
      | plot([xrad -x x xrad], [yrad -y y yrad]);
      | fprintf('NI Out%d', portnum);
  wires:
  In1/1 -> Test_KeyPostn_No/1
  In2/1 -> Test_Te50/1
  In3/1 -> Test_Te15/1
  In4/1 -> Test_KVactive/1
  In5/1 -> Test_ClutchSW/1
  In6/1 -> Test_PCMWakeup/1

== system P702_NI_SoftECU/SoftECU/PCM/Mapping/EngineData_7/Count ==
  Stepsize : Inport
  MaxValue : Inport  Port=2
  Reset : Inport  Port=3
  Enable : EnablePort
  Gain : Gain  Gain=1000
  Integrator1 : Integrator  ExternalReset=rising  InitialConditionSource=external
  Math Function : Math  Operator=mod  SaturateOnIntegerOverflow=on
  Product : Product  RndMeth=Zero
  Relational Operator : RelationalOperator  Operator=<  OutDataTypeStr=boolean  RndMeth=Nearest
  Sum1 : Sum  Inputs=|++
  Xo1 : Constant  Value=0
  offset : Constant
  OdoCount : Outport
  OverallCount : Outport  Port=2
  wires:
  Product/1 -> OdoCount/1
  Relational Operator/1 -> Product/2
  Sum1/1 -> Math Function/2
  MaxValue/1 -> Relational Operator/2, Sum1/1
  offset/1 -> Sum1/2
  Math Function/1 -> Product/1, Relational Operator/1
  Xo1/1 -> Integrator1/3
  Integrator1/1 -> Math Function/1, OverallCount/1
  Reset/1 -> Integrator1/2
  Stepsize/1 -> Gain/1
  Gain/1 -> Integrator1/1

== system P702_NI_SoftECU/SoftECU/PCM/Mapping/EngineData_7/Count1 ==
  Stepsize : Inport
  MaxValue : Inport  Port=2
  Reset : Inport  Port=3
  Enable : EnablePort
  Gain : Gain  Gain=1000
  Integrator1 : Integrator  ExternalReset=rising  InitialConditionSource=external
  Math Function : Math  Operator=mod  SaturateOnIntegerOverflow=on
  Sum1 : Sum  Inputs=|++
  Xo1 : Constant  Value=0
  offset : Constant  Value=0
  OdoCount : Outport
  OverallCount : Outport  Port=2
  wires:
  Sum1/1 -> Math Function/2
  MaxValue/1 -> Sum1/1
  offset/1 -> Sum1/2
  Math Function/1 -> OdoCount/1
  Xo1/1 -> Integrator1/3
  Integrator1/1 -> Math Function/1, OverallCount/1
  Reset/1 -> Integrator1/2
  Stepsize/1 -> Gain/1
  Gain/1 -> Integrator1/1

== system P702_NI_SoftECU/SoftECU/PCM/Mapping/EngineData_7/FuelFlw_Vl_Dsply ==
  Enable : Inport
  Trigger : Inport  Port=2
  MsgCycleTime : Inport  Port=3
  NumberOfCounts : Inport  Port=4
  Runtime : Inport  Port=5
  Reset : Inport  Port=6
  Constant : Constant  Value=1024
  Constant1 : Constant  Value=1024
  Constant4 : Constant
  Count : Subsystem
  Detect Increase : simulink/Logic and Bit Operations/Detect Increase  vinit=0.0  OutDataTypeStr=boolean
  Detect Increase1 : simulink/Logic and Bit Operations/Detect Increase  vinit=0.0  OutDataTypeStr=boolean
  Divide : Product  Inputs=*/*
  Divide1 : Product  Inputs=*/
  Logical Operator : Logic  Inputs=3  AllPortsSameDT=off  OutDataTypeStr=boolean
  Logical Operator1 : Logic  Operator=OR  AllPortsSameDT=off  OutDataTypeStr=boolean
  Logical Operator2 : Logic  Operator=OR  AllPortsSameDT=off  OutDataTypeStr=boolean
  Rounding Function : Rounding
  Rounding Function1 : Rounding
  Timer : Subsystem
  StepSize : Outport
  CAN_signal : Outport  Port=2
  OverallCount : Outport  Port=3
  ElapsedTime : Outport  Port=4
  NumPeriods : Outport  Port=5
  wires:
  Rounding Function1/1 -> OverallCount/1
  Rounding Function/1 -> CAN_signal/1
  Logical Operator2/1 -> Count/Enable
  Logical Operator/1 -> Logical Operator2/2
  Logical Operator1/1 -> Logical Operator2/1, Timer/3(Reset), Count/3(Reset)
  Detect Increase1/1 -> Logical Operator1/2
  Detect Increase/1 -> Logical Operator1/1
  Reset/1 -> Detect Increase1/1
  Divide1/1 -> NumPeriods/1
  Constant1/1 -> Divide1/2
  MsgCycleTime/1 -> Divide/3
  Trigger/1 -> Logical Operator/1
  NumberOfCounts/1 -> Divide1/1, Divide/1
  Timer/2(ElapsedTime) -> ElapsedTime/1
  Count/2(OverallCount) -> Rounding Function1/1
  Count/1(OdoCount) -> Rounding Function/1
  Divide/1 -> Count/1(Stepsize), StepSize/1
  Timer/1(Active) -> Logical Operator/3
  Constant/1 -> Count/2(MaxValue)
  Runtime/1 -> Timer/2(Runtime), Divide/2
  Enable/1 -> Timer/Enable, Logical Operator/2, Detect Increase/1
  Constant4/1 -> Timer/1(Stepsize)

== system P702_NI_SoftECU/SoftECU/PCM/Mapping/EngineData_7/ODoCount ==
  Enable : Inport
  Trigger : Inport  Port=2
  MsgCycleTime : Inport  Port=3
  NumberOfCounts : Inport  Port=4
  Runtime : Inport  Port=5
  Reset : Inport  Port=6
  Constant : Constant  Value=255
  Constant1 : Constant  Value=256
  Constant4 : Constant
  Count : Subsystem
  Detect Increase : simulink/Logic and Bit Operations/Detect Increase  vinit=0.0  OutDataTypeStr=boolean
  Detect Increase1 : simulink/Logic and Bit Operations/Detect Increase  vinit=0.0  OutDataTypeStr=boolean
  Divide : Product  Inputs=*/*
  Divide1 : Product  Inputs=*/
  Logical Operator : Logic  Inputs=3  AllPortsSameDT=off  OutDataTypeStr=boolean
  Logical Operator1 : Logic  Operator=OR  AllPortsSameDT=off  OutDataTypeStr=boolean
  Logical Operator2 : Logic  Operator=OR  AllPortsSameDT=off  OutDataTypeStr=boolean
  Rounding Function : Rounding
  Rounding Function1 : Rounding
  Timer : Subsystem
  StepSize : Outport
  CAN_signal : Outport  Port=2
  OverallCount : Outport  Port=3
  ElapsedTime : Outport  Port=4
  NumPeriods : Outport  Port=5
  wires:
  Rounding Function1/1 -> OverallCount/1
  Rounding Function/1 -> CAN_signal/1
  Logical Operator2/1 -> Count/Enable
  Logical Operator/1 -> Logical Operator2/2
  Logical Operator1/1 -> Logical Operator2/1, Timer/3(Reset), Count/3(Reset)
  Detect Increase1/1 -> Logical Operator1/2
  Detect Increase/1 -> Logical Operator1/1
  Reset/1 -> Detect Increase1/1
  Divide1/1 -> NumPeriods/1
  Constant1/1 -> Divide1/2
  MsgCycleTime/1 -> Divide/3
  Trigger/1 -> Logical Operator/1
  NumberOfCounts/1 -> Divide1/1, Divide/1
  Timer/2(ElapsedTime) -> ElapsedTime/1
  Count/2(OverallCount) -> Rounding Function1/1
  Count/1(OdoCount) -> Rounding Function/1
  Divide/1 -> Count/1(Stepsize), StepSize/1
  Timer/1(Active) -> Logical Operator/3
  Constant/1 -> Count/2(MaxValue)
  Runtime/1 -> Timer/2(Runtime), Divide/2
  Enable/1 -> Timer/Enable, Logical Operator/2, Detect Increase/1
  Constant4/1 -> Timer/1(Stepsize)

== system P702_NI_SoftECU/SoftECU/PCM/Mapping/EngineData_7/scaling ==
  In1 : Inport
  kmh_ms : Gain  Gain=1/3.6
  m_2_count : Gain  Gain=1/0.2
  ms_m0.1s : Gain  Gain=0.1
  Out1 : Outport
  wires:
  m_2_count/1 -> Out1/1
  ms_m0.1s/1 -> m_2_count/1
  In1/1 -> kmh_ms/1
  kmh_ms/1 -> ms_m0.1s/1

== system P702_NI_SoftECU/SoftECU/PCM/Mapping/EngineData_7/scaling_ ==
  FuelFlw_Vl_DsplyStep_No : Constant
  µl_2_count : Gain  Gain=1/25
  Out1 : Outport
  wires:
  µl_2_count/1 -> Out1/1
  FuelFlw_Vl_DsplyStep_No/1 -> µl_2_count/1

== system P702_NI_SoftECU/SoftECU/SCCM/Logic/Map_Inputs/Maneuver ==
  ECU_Commands[] : Inport
  Reset[0|1] : Inport  Port=2
  Add : Sum  Inputs=+++
  Constant : Constant
  Fcn1 : Fcn  Expr=u(1)==1020
  Fcn10 : Fcn  Expr=u(1)==1031
  Fcn2 : Fcn  Expr=u(1)==1030
  Fcn3 : Fcn  Expr=u(1)==1022
  Fcn4 : Fcn  Expr=u(1)==1021
  Fcn5 : Fcn  Expr=u(1)==1013
  Fcn6 : Fcn  Expr=u(1)==1011
  Fcn7 : Fcn  Expr=u(1)==1010
  Fcn8 : Fcn  Expr=u(1)==1012
  Fcn9 : Fcn  Expr=u(1)==1032
  Gain : Gain
  Gain1 : Gain  Gain=2
  Gain2 : Gain  Gain=3
  Logical Operator : Logic  Operator=OR  Inputs=4  AllPortsSameDT=off  OutDataTypeStr=boolean
  Memory : Memory  InitialCondition=1
  Switch : Switch  Threshold=0.5
  Switch1 : Switch  Threshold=0.5
  pos_edge_detection : Subsystem
  pos_edge_detection1 : Subsystem
  pos_edge_detection2 : Subsystem
  pos_edge_detection3 : Subsystem
  Sw_ACC_On[0Off|1On] : Outport
  Sw_ACC_Off[0Off|1On] : Outport  Port=2
  Sw_ACC_Cancel[0Off|1On] : Outport  Port=3
  Sw_ACC_Resume[0Off|1On] : Outport  Port=4
  Sw_ACC_Speed_Set[0Off|1On] : Outport  Port=5
  Sw_ACC_Speed_Increase[0Off|1On] : Outport  Port=6
  Sw_ACC_Speed_Decrease[0Off|1On] : Outport  Port=7
  Sw_ACC_BrakeMode[1Comfort|2AEBOnly|3AEBOff] : Outport  Port=8
  wires:
  Constant/1 -> Switch1/1
  Switch1/1 -> Switch/1
  Reset[0|1]/1 -> pos_edge_detection3/1(In1)
  Add/1 -> Switch1/3
  pos_edge_detection3/1(Out1) -> Logical Operator/4, Switch1/2
  Memory/1 -> Switch/3
  Switch/1 -> Memory/1, Sw_ACC_BrakeMode[1Comfort|2AEBOnly|3AEBOff]/1
  Logical Operator/1 -> Switch/2
  Gain/1 -> Add/1
  Gain1/1 -> Add/2
  Gain2/1 -> Add/3
  pos_edge_detection2/1(Out1) -> Logical Operator/3
  pos_edge_detection1/1(Out1) -> Logical Operator/2
  pos_edge_detection/1(Out1) -> Logical Operator/1
  Fcn2/1 -> Gain/1, pos_edge_detection2/1(In1)
  Fcn10/1 -> Gain1/1, pos_edge_detection1/1(In1)
  Fcn9/1 -> Gain2/1, pos_edge_detection/1(In1)
  ECU_Commands[]/1 -> Fcn3/1, Fcn2/1, Fcn10/1, Fcn9/1, Fcn4/1, Fcn1/1, Fcn5/1, Fcn8/1, Fcn6/1, Fcn7/1
  Fcn1/1 -> Sw_ACC_Speed_Set[0Off|1On]/1
  Fcn8/1 -> Sw_ACC_Cancel[0Off|1On]/1
  Fcn5/1 -> Sw_ACC_Resume[0Off|1On]/1
  Fcn4/1 -> Sw_ACC_Speed_Increase[0Off|1On]/1
  Fcn3/1 -> Sw_ACC_Speed_Decrease[0Off|1On]/1
  Fcn7/1 -> Sw_ACC_On[0Off|1On]/1
  Fcn6/1 -> Sw_ACC_Off[0Off|1On]/1

== system P702_NI_SoftECU/SoftECU/SRR_L/FrontLeft_SOD/SRR_FL_001/Subsystem ==
  target_pos : Inport
  sensor_pos : Inport  Port=2
  CSP : Inport  Port=3
  Abs : Abs
  Add : Sum  Inputs=++-+
  Add1 : Sum  Inputs=++-+
  Add2 : Sum  Inputs=+-
  Add3 : Sum
  Bus Selector : BusSelector  OutputSignals=SRR_L_DET_RANGE_01[m],SRR_L_DET_AZIMUTH_01[rad],SRR_L_DET_RANGE_RATE_01[m/s],SRR_L_DET_ELEVATION_01[rad]
  Bus Selector1 : BusSelector  OutputSignals=sensor_x,sensor_y,sensor_yaw
  Bus Selector2 : BusSelector  OutputSignals=c_sensor_x,c_sensor_y,c_sensor_yaw
  Constant : Constant
  Index Vector : MultiPortSwitch  DataPortOrder=Zero-based contiguous  Inputs=2  zeroidx=on
  Index Vector1 : MultiPortSwitch  DataPortOrder=Zero-based contiguous  Inputs=2  zeroidx=on
  Logical Operator : Logic  AllPortsSameDT=off  OutDataTypeStr=boolean
  Math Function : Math  Operator=magnitude^2  SaturateOnIntegerOverflow=on
  Math Function1 : Math  Operator=magnitude^2  SaturateOnIntegerOverflow=on
  Product : Product
  Product1 : Product
  Product2 : Product
  Relational Operator : RelationalOperator  Operator=<=  OutDataTypeStr=boolean  RndMeth=Simplest
  Relational Operator1 : RelationalOperator  Operator=<=  OutDataTypeStr=boolean  RndMeth=Simplest
  Sqrt : Sqrt  SaturateOnIntegerOverflow=on
  Terminator : Terminator
  atan_cal : Trigonometry  Operator=atan2
  atan_cal1 : Trigonometry  Operator=atan2
  not_valid_azimuth : Constant  Value=0
  not_valid_range : Constant  Value=-1
  random_factor : Subsystem
  random_factor1 : Subsystem
  sincal : Trigonometry
  sincal1 : Trigonometry  Operator=cos
  sincal2 : Trigonometry
  sincal3 : Trigonometry  Operator=cos
  range : Outport
  range_rate : Outport  Port=2
  azimuth : Outport  Port=3
  elevation : Outport  Port=4
  wires:
  random_factor1/1(Rand_Error) -> Add1/4
  random_factor/1(Rand_Error) -> Add/4
  [AngleScanRange] -> Relational Operator1/2
  [DistanceScanRange] -> Relational Operator/2
  Abs/1 -> Relational Operator1/1
  Add2/1 -> sincal2/1, sincal3/1
  sincal3/1 -> atan_cal1/2
  sincal2/1 -> atan_cal1/1
  atan_cal1/1 -> Product2/1
  not_valid_azimuth/1 -> Index Vector1/2
  Logical Operator/1 -> Index Vector/1, Index Vector1/1
  Index Vector1/1 -> azimuth/1
  not_valid_range/1 -> Index Vector/2
  Index Vector/1 -> range/1
  Relational Operator1/1 -> Logical Operator/2
  Relational Operator/1 -> Logical Operator/1
  Product2/1 -> Index Vector1/3, Abs/1
  Sqrt/1 -> Relational Operator/1, Index Vector/3
  Bus Selector/4 -> elevation/1  "<SRR_L_DET_ELEVATION_01[rad]>"
  Bus Selector/3 -> range_rate/1  "<SRR_L_DET_RANGE_RATE_01[m/s]>"
  Constant/1 -> Product2/2
  Add3/1 -> Sqrt/1
  Math Function1/1 -> Add3/2
  Math Function/1 -> Add3/1
  atan_cal/1 -> Add2/1
  Add1/1 -> atan_cal/2, Math Function1/1
  Add/1 -> atan_cal/1, Math Function/1
  Product1/1 -> Add1/1
  Bus Selector1/3 -> Add2/2  "<sensor_yaw>"
  Bus Selector1/2 -> Add/3  "<sensor_y>"
  Bus Selector1/1 -> Add1/3  "<sensor_x>"
  Bus Selector2/3 -> Terminator/1  "<c_sensor_yaw>"
  Bus Selector2/2 -> Add/2  "<c_sensor_y>"
  Bus Selector2/1 -> Add1/2  "<c_sensor_x>"
  CSP/1 -> Bus Selector2/1
  sensor_pos/1 -> Bus Selector1/1
  Product/1 -> Add/1
  sincal1/1 -> Product1/2
  sincal/1 -> Product/2
  Bus Selector/2 -> sincal/1, sincal1/1  "<SRR_L_DET_AZIMUTH_01[rad]>"
  Bus Selector/1 -> Product/1, Product1/1, random_factor1/1(Range), random_factor/1(Range)  "<SRR_L_DET_RANGE_01[m]>"
  target_pos/1 -> Bus Selector/1
